simulink model "primerito"  (R2023a)
settings: Solver=VariableStepAuto  StartTime=0.0  StopTime=50  RelTol=1e-3
undefined symbols (not defined in the file): m, n
settings Model: Creator=Celia Hermana  LastModifiedBy=santi

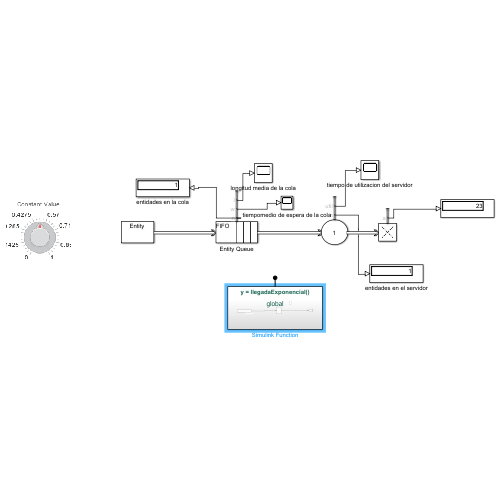
[thumbnail: Simulink's stored preview of the top-level diagram]
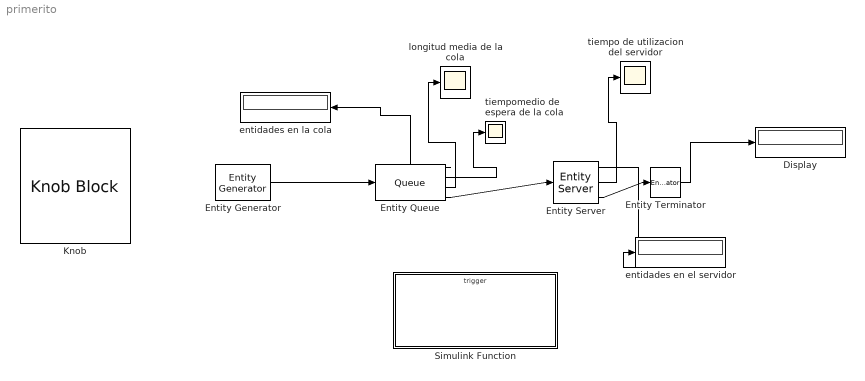
== system primerito ==
  Display : Display
  Entity Generator : EntityGenerator  OutputPortMessageModes=m  TimeSource=MATLAB action  IntergenerationTimeAction=dt = llegadaExponencial();  EntityType=Structured  EntityTypeName=Entity
  Entity Queue : Queue  InputPortMessageModes=m  OutputPortMessageModes=n,n,n,m  Capacity=500  NumberEntitiesInBlock=on  AverageWait=on  AverageQueueLength=on
      settings: OutputPortMap=o1,o2,o3,o5
  Entity Server : EntityServer  InputPortMessageModes=m  OutputPortMessageModes=n,n,m  Capacity=1  ServiceTimeSource=MATLAB action  ServiceTimeAction=|  NumberEntitiesInBlock=on  Utilization=on
      | media = 1
      | dt = -media*log(1-rand());
      settings: OutputPortMap=o1,o5,o9
  Entity Terminator : EntityTerminator  InputPortMessageModes=m  NumberEntitiesArrived=on
      settings: OutputPortMap=o0
  Knob : KnobBlock  ScaleMax=1
  Simulink Function : Subsystem  TreatAsAtomicUnit=on
  entidades en el servidor : Display
  entidades en la cola : Display
  longitud media de la cola : Scope
  tiempo de utilizacion del servidor : Scope
  tiempomedio de espera de la cola : Scope
  wires:
  Entity Generator/1 -> Entity Queue/1
  Entity Queue/4 -> Entity Server/1
  Entity Server/3 -> Entity Terminator/1
  Entity Queue/3 -> longitud media de la cola/1
  Entity Queue/2 -> tiempomedio de espera de la cola/1
  Entity Server/2 -> tiempo de utilizacion del servidor/1
  Entity Terminator/1 -> Display/1
  Entity Queue/1 -> entidades en la cola/1
  Entity Server/1 -> entidades en el servidor/1

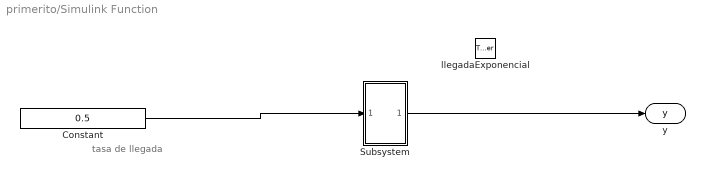
== system primerito/Simulink Function ==
  note: tasa de llegada
  llegadaExponencial : TriggerPort  TriggerType=function-call  IsSimulinkFunction=on  FunctionName=llegadaExponencial  VariantControl=(inherit)
  Constant : Constant  Value=0.5
  Subsystem : Subsystem
  y : ArgOut  DisableCoverage=on  ArgumentName=y
  wires:
  Constant/1 -> Subsystem/1(In1)
  Subsystem/1(Out1) -> y/1

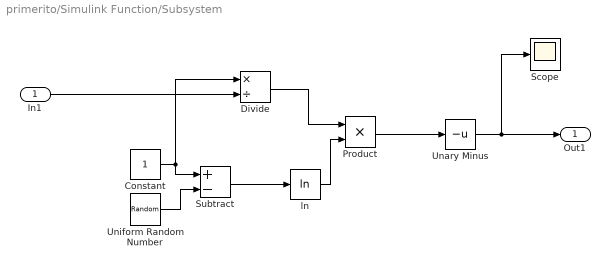
== system primerito/Simulink Function/Subsystem ==
  In1 : Inport
  Constant : Constant
  Divide : Product  Inputs=*/
  Product : Product
  Scope : Scope
  Subtract : Sum  Inputs=+-
  Unary Minus : UnaryMinus
  Uniform Random Number : UniformRandomNumber  Minimum=0  Seed=12345
  ln : Math  Operator=log
  Out1 : Outport
  wires:
  Uniform Random Number/1 -> Subtract/2
  ln/1 -> Product/2
  In1/1 -> Divide/2
  Product/1 -> Unary Minus/1
  Divide/1 -> Product/1
  Constant/1 -> Subtract/1, Divide/1
  Subtract/1 -> ln/1
  Unary Minus/1 -> Scope/1, Out1/1
